simulink model "W06_3_heading_offline"  (R2024b)
settings: Solver=ode4  StartTime=0.0  StopTime=40  FixedStep=0.05  RelTol=1e-3
settings Model: Creator=admin  LastModifiedBy=admin

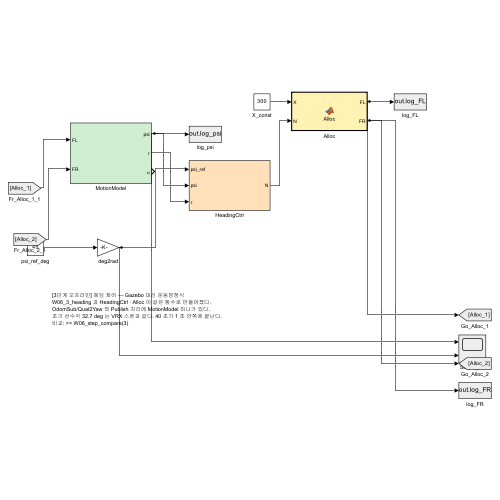
[thumbnail: Simulink's stored preview of the top-level diagram]
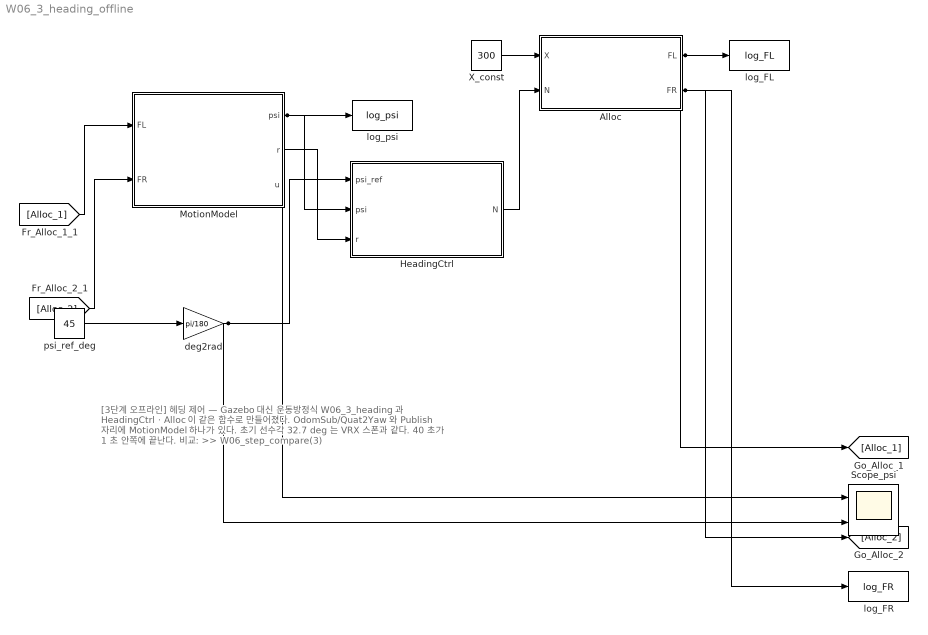
== system W06_3_heading_offline ==
  note: [3단계 오프라인] 헤딩 제어 — Gazebo 대신 운동방정식
      | W06_3_heading 과 HeadingCtrl · Alloc 이 같은 함수로 만들어졌다.
      | OdomSub/Quat2Yaw 와 Publish 자리에 MotionModel 하나가 있다.
      | 초기 선수각 32.7 deg 는 VRX 스폰과 같다. 40 초가 1 초 안쪽에 끝난다.
      | 비교: >> W06_step_compare(3)
  Alloc : MATLAB Function  TreatAsAtomicUnit=on
  HeadingCtrl : Subsystem
  MotionModel : Subsystem
  Scope_psi : Scope  NumInputPorts=2
  X_const : Constant  Value=300
  deg2rad : Gain  Gain=pi/180
  log_FL : ToWorkspace  VariableName=log_FL  SaveFormat=Timeseries  SampleTime=0.05
  log_FR : ToWorkspace  VariableName=log_FR  SaveFormat=Timeseries  SampleTime=0.05
  log_psi : ToWorkspace  VariableName=log_psi  SaveFormat=Timeseries  SampleTime=0.05
  psi_ref_deg : Constant  Value=45
  wires:
  psi_ref_deg/1 -> deg2rad/1
  MotionModel/1(psi) -> HeadingCtrl/2(psi), log_psi/1, Scope_psi/1
  MotionModel/2(r) -> HeadingCtrl/3(r)
  X_const/1 -> Alloc/1(X)
  deg2rad/1 -> HeadingCtrl/1(psi_ref), Scope_psi/2
  HeadingCtrl/1(N) -> Alloc/2(N)
  Alloc/1(FL) -> log_FL/1, [Alloc_1]
  [Alloc_2] -> MotionModel/2(FR)
  Alloc/2(FR) -> [Alloc_2], log_FR/1
  [Alloc_1] -> MotionModel/1(FL)

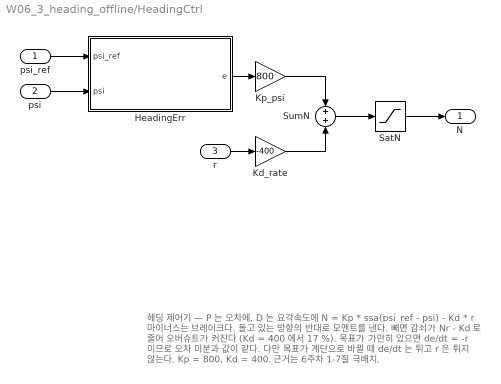
== system W06_3_heading_offline/HeadingCtrl ==
  note: 헤딩 제어기 — P 는 오차에, D 는 요각속도에
      |
      |     N = Kp * ssa(psi_ref - psi)  -  Kd * r
      |
      | 마이너스는 브레이크다. 돌고 있는 방향의 반대로 모멘트를 낸다.
      | 빼면 감쇠가 Nr - Kd 로 줄어 오버슈트가 커진다 (Kd = 400 에서 17 %).
      |
      | 목표가 가만히 있으면 de/dt = -r 이므로 오차 미분과 값이 같다.
      | 다만 목표가 계단으로 바뀔 때 de/dt 는 튀고 r 은 튀지 않는다.
      |
      | Kp = 800, Kd = 400.  근거는 6주차 1-7절 극배치.
  psi_ref : Inport
  psi : Inport  Port=2
  r : Inport  Port=3
  HeadingErr : MATLAB Function  TreatAsAtomicUnit=on
  Kd_rate : Gain  Gain=-400
  Kp_psi : Gain  Gain=800
  SatN : Saturate  UpperLimit=500  LowerLimit=-500
  SumN : Sum
  N : Outport
  wires:
  psi_ref/1 -> HeadingErr/1(psi_ref)
  psi/1 -> HeadingErr/2(psi)
  Kd_rate/1 -> SumN/2
  HeadingErr/1(e) -> Kp_psi/1
  SatN/1 -> N/1
  r/1 -> Kd_rate/1
  SumN/1 -> SatN/1
  Kp_psi/1 -> SumN/1

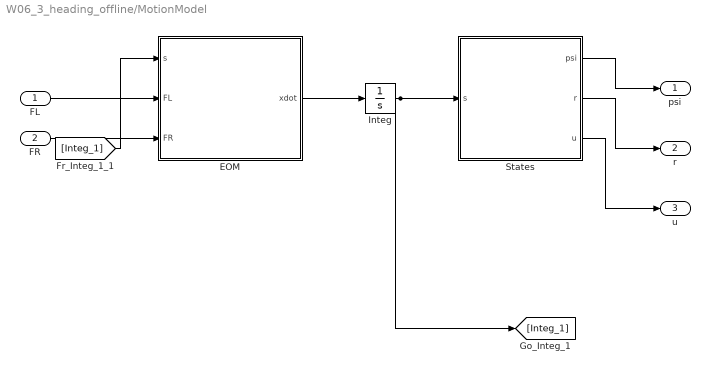
== system W06_3_heading_offline/MotionModel ==
  FL : Inport
  FR : Inport  Port=2
  EOM : MATLAB Function  TreatAsAtomicUnit=on
  Integ : Integrator  InitialCondition=[0;0;0;0;0;32.7*pi/180]
  States : MATLAB Function  TreatAsAtomicUnit=on
  psi : Outport
  r : Outport  Port=2
  u : Outport  Port=3
  wires:
  FL/1 -> EOM/2(FL)
  FR/1 -> EOM/3(FR)
  EOM/1(xdot) -> Integ/1
  Integ/1 -> States/1(s), [Integ_1]
  States/1(psi) -> psi/1
  States/2(r) -> r/1
  States/3(u) -> u/1
  [Integ_1] -> EOM/1(s)

== matlab function W06_3_heading_offline/MotionModel/EOM ==
  data: s input; xdot output; FL input; FR input
function xdot = EOM(s, FL, FR)
%#codegen
% 3-DOF WAM-V equations of motion, NED (3주차 1-8 절).
%   s = [u v r x_n y_n psi]'
m = 211;  Izz = 653;  Xu = 100;  Xuu = 150;  Yv = 100;  Yvv = 100;
Nr = 800;  Nrr = 800;  b_half = 1.027135;
u = s(1); v = s(2); r = s(3); psi = s(6);
X = FL + FR;
N = (FL - FR)*b_half;
du = (X - (Xu + Xuu*abs(u))*u)/m + v*r;
dv = (  - (Yv + Yvv*abs(v))*v)/m - u*r;
dr = (N - (Nr + Nrr*abs(r))*r)/Izz;
xdot = [du; dv; dr;
        u*cos(psi) - v*sin(psi);
        u*sin(psi) + v*cos(psi);
        r];

== matlab function W06_3_heading_offline/HeadingCtrl/HeadingErr ==
  data: psi_ref input; e output; psi input
function e = HeadingErr(psi_ref, psi)
%#codegen
% Shortest signed angle, wrapped to [-pi, pi]
d = psi_ref - psi;
e = atan2(sin(d), cos(d));

== matlab function W06_3_heading_offline/Alloc ==
  data: X input; FL output; N input; FR output
function [FL, FR] = Alloc(X, N)
%#codegen
% Differential thrust allocation for the 2-thruster WAM-V
%   X : surge force  [N]
%   N : yaw moment   [N*m], positive turns to starboard
B_half = 1.027135;      % half distance between thrusters [m]
Fmax   = 250;           % thrust limit per thruster [N]
FL = X/2 + N/(2*B_half);
FR = X/2 - N/(2*B_half);
FL = max(min(FL, Fmax), -Fmax);
FR = max(min(FR, Fmax), -Fmax);

== matlab function W06_3_heading_offline/MotionModel/States ==
  data: s input; psi output; r output; u output
function [psi, r, u] = States(s)
%#codegen
% Quat2Yaw 와 같은 출력 — 선수각은 [-pi, pi] 로 접는다
psi = atan2(sin(s(6)), cos(s(6)));
r = s(3);
u = s(1);
